simulink model "chatter_with_subsystem"  (R2013a)
settings: Solver=ode45  StartTime=0.0  StopTime=100.0  RelTol=1e-3
PreLoadFcn:
  | m=10
  | g=9.8
  | N=g*m
  | k=100
  | mu=.3
  | v=.3
  | zv=v/1000
PostLoadFcn:
  | plot(1:10)
libraries: simulink x1
settings Model: Creator=macuser  LastModifiedBy=macuser

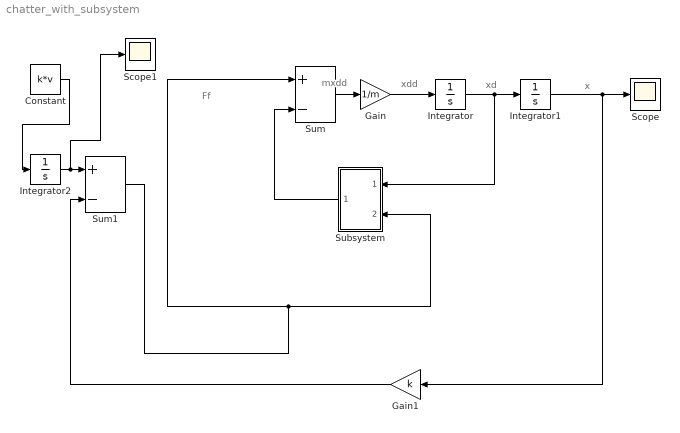
== system chatter_with_subsystem ==
  note: Ff
  note: x
  note: xd
  note: xdd
  note: mxdd
  Constant : Constant  Value=k*v
  Gain : Gain  Gain=1/m
  Gain1 : Gain  Gain=k
  Integrator : Integrator
  Integrator1 : Integrator
  Integrator2 : Integrator
  Scope : Scope
  Scope1 : Scope
  Subsystem : Subsystem
  Sum : Sum  Inputs=+-
  Sum1 : Sum  Inputs=+-
  wires:
  Sum/1 -> Gain/1
  Gain/1 -> Integrator/1
  Integrator/1 -> Subsystem/1(In1), Integrator1/1
  Integrator1/1 -> Gain1/1, Scope/1
  Constant/1 -> Integrator2/1
  Integrator2/1 -> Scope1/1, Sum1/1
  Gain1/1 -> Sum1/2
  Sum1/1 -> Subsystem/2(In2), Sum/1
  Subsystem/1(Out1) -> Sum/2

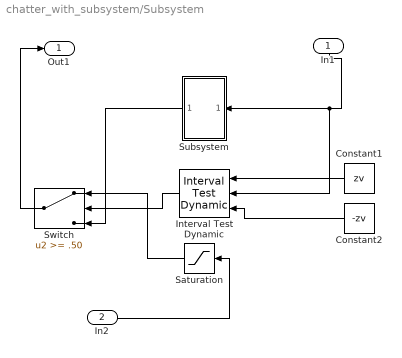
== system chatter_with_subsystem/Subsystem ==
  In1 : Inport
  In2 : Inport  Port=2
  Constant1 : Constant  Value=zv
  Constant2 : Constant  Value=-zv
  Interval Test Dynamic : simulink/Logic and Bit Operations/Interval Test Dynamic  IntervalClosedRight=on  IntervalClosedLeft=on  OutDataTypeStr=uint8
  Saturation : Saturate  UpperLimit=mu*N  LowerLimit=-mu*N
  Subsystem : Subsystem
  Switch : Switch  Threshold=.50
  Out1 : Outport
  wires:
  Switch/1 -> Out1/1
  Saturation/1 -> Switch/1
  Constant2/1 -> Interval Test Dynamic/3
  Constant1/1 -> Interval Test Dynamic/1
  Interval Test Dynamic/1 -> Switch/2
  In1/1 -> Subsystem/1(In1), Interval Test Dynamic/2
  In2/1 -> Saturation/1
  Subsystem/1(Out1) -> Switch/3

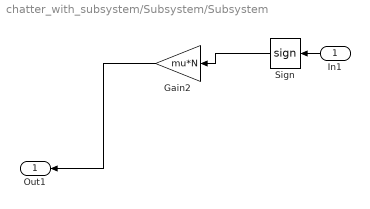
== system chatter_with_subsystem/Subsystem/Subsystem ==
  In1 : Inport
  Gain2 : Gain  Gain=mu*N
  Sign : Signum
  Out1 : Outport
  wires:
  Sign/1 -> Gain2/1
  Gain2/1 -> Out1/1
  In1/1 -> Sign/1
